simulink model "UAM_FlightModeManager"  (R2024b)
settings: Solver=VariableStepAuto  StartTime=0.0  StopTime=10.0  RelTol=1e-3
settings Model: DataDictionary=UAM_data.sldd  Creator=admin  LastModifiedBy=USER

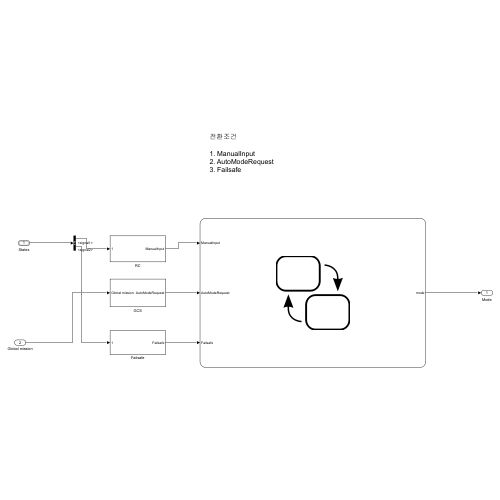
[thumbnail: Simulink's stored preview of the top-level diagram]
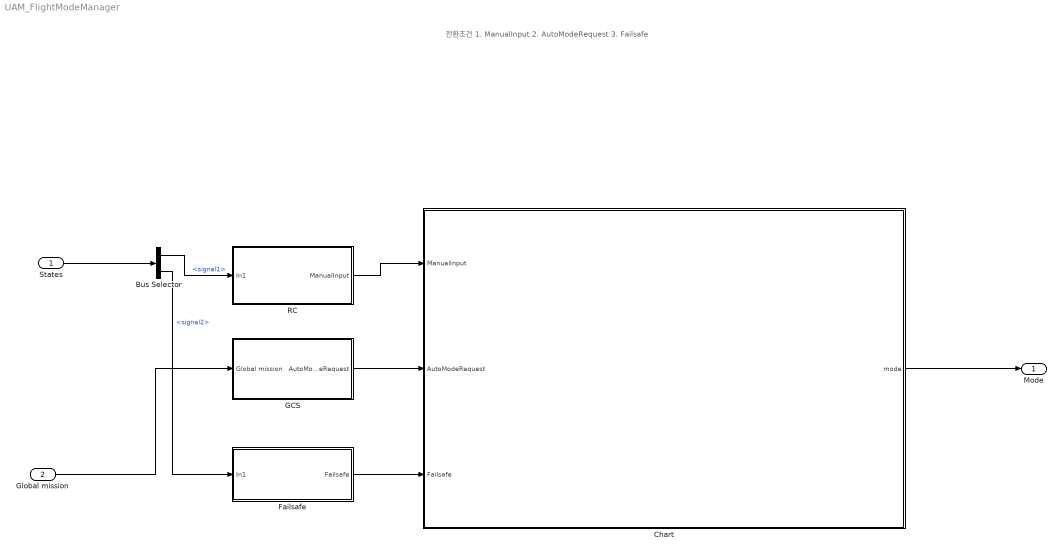
== system UAM_FlightModeManager ==
  note: 전환조건
      |
      | 1. ManualInput
      | 2. AutoModeRequest
      | 3. Failsafe
  States : Inport  OutDataTypeStr=Bus: StateBus
  Global mission : Inport  Port=2
  Bus Selector : BusSelector  OutputSignals=signal1,signal2
  Chart : Stateflow chart  TreatAsAtomicUnit=on
  Failsafe : Subsystem
  GCS : Subsystem
  RC : Subsystem
  Mode : Outport
  wires:
  States/1 -> Bus Selector/1
  Chart/1(mode) -> Mode/1
  Global mission/1 -> GCS/1(Global mission)
  Bus Selector/2 -> Failsafe/1(In1)  "<signal2>"
  Bus Selector/1 -> RC/1(In1)  "<signal1>"
  RC/1(ManualInput) -> Chart/1(ManualInput)
  GCS/1(AutoModeRequest) -> Chart/2(AutoModeRequest)
  Failsafe/1(Failsafe) -> Chart/3(Failsafe)

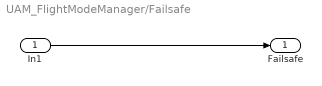
== system UAM_FlightModeManager/Failsafe ==
  In1 : Inport
  Failsafe : Outport
  wires:
  In1/1 -> Failsafe/1

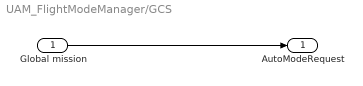
== system UAM_FlightModeManager/GCS ==
  Global mission : Inport
  AutoModeRequest : Outport
  wires:
  Global mission/1 -> AutoModeRequest/1

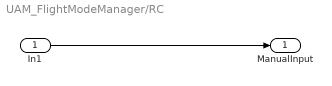
== system UAM_FlightModeManager/RC ==
  In1 : Inport
  ManualInput : Outport
  wires:
  In1/1 -> ManualInput/1

== stateflow chart UAM_FlightModeManager/Chart ==
  state Manual
    Mode = FlightModeType.Manual;
  state Auto
    Mode = FlightModeType.Auto;
  state Emergency
    Mode = FlightModeType.Emergency;
  (default) -> Manual
  Manual -> Auto [order 1] : [AutoModeRequest && ~Failsafe]
  Auto -> Manual [order 1] : [ManualInput && ~Failsafe]
  Manual -> Emergency [order 2] : [Failsafe]
  Emergency -> Manual [order 1] : [[ManualInput && ~Failsafe]]
  Auto -> Emergency [order 2] : [Failsafe]
  Emergency -> Auto [order 2] : [[AutoModeRequest && ~Failsafe]]
  data: ManualInput input boolean; AutoModeRequest input boolean; Failsafe input boolean; mode output Enum: FlightModeType
